simulink model "loadSimulator"  (R2025b)
settings: Solver=VariableStepAuto  StartTime=0.0  StopTime=50  RelTol=1e-3
values from neighbouring files (symbols this model uses):
  xL0 = [0.8;0.8;0.1]    [parametrosCarga4x.m]
settings Model: Creator=ateveraz  LastModifiedBy=ateveraz

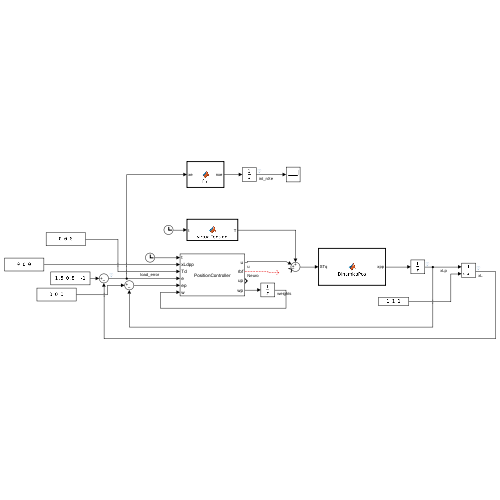
[thumbnail: Simulink's stored preview of the top-level diagram]
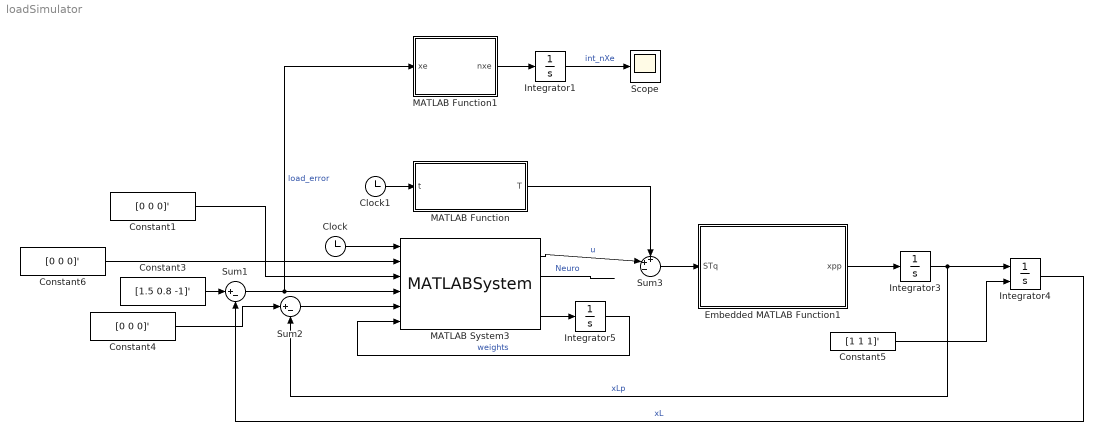
== system loadSimulator ==
  Clock : Clock
  Clock1 : Clock
  Constant1 : Constant  Value=[0 0 0]'
  Constant3 : Constant  Value=[1.5 0.8 -1]'
  Constant4 : Constant  Value=[0 0 0]'
  Constant5 : Constant  Value=[1 1 1]'
  Constant6 : Constant  Value=[0 0 0]'
  Embedded MATLAB Function1 : MATLAB Function  TreatAsAtomicUnit=on
  Integrator1 : Integrator
  Integrator3 : Integrator  InitFcn=parametrosCarga4x  InitialCondition=[0;0;0]
  Integrator4 : Integrator  InitFcn=parametrosCarga4x  InitialConditionSource=external  InitialCondition=xL0
  Integrator5 : Integrator  InitialCondition=zeros(3,15)
  MATLAB Function : MATLAB Function  TreatAsAtomicUnit=on
  MATLAB Function1 : MATLAB Function  TreatAsAtomicUnit=on
  MATLAB System3 : MATLABSystem  System=PositionController  Kd=2.0  alpha=1.0  mass=-0.225  Gamma=0.1  kappa=0.01  k=10  N_neurons=15  center_range=1.0  eta_width=1.5  SimulateUsing=Code generation
      mask Type: PositionController
  Scope : Scope
      settings: ActiveDisplayYMinimum=-1  ActiveDisplayYMaximum=1
  Sum1 : Sum  Inputs=|+-
  Sum2 : Sum  Inputs=|+-
  Sum3 : Sum  Inputs=++-|
  wires:
  Constant3/1 -> Sum1/1
  Sum1/1 -> MATLAB Function1/1(xe), MATLAB System3/4  "load_error"
  Sum2/1 -> MATLAB System3/5
  Constant4/1 -> Sum2/1
  Embedded MATLAB Function1/1(xpp) -> Integrator3/1
  Constant5/1 -> Integrator4/2
  Integrator3/1 -> Integrator4/1, Sum2/2  "xLp"
  Integrator4/1 -> Sum1/2  "xL"
  Sum3/1 -> Embedded MATLAB Function1/1(STq)
  MATLAB System3/2 -> ?  "Neuro"
  MATLAB System3/1 -> Sum3/2  "u"
  Constant6/1 -> MATLAB System3/2
  Clock/1 -> MATLAB System3/1
  MATLAB System3/4 -> Integrator5/1
  Integrator5/1 -> MATLAB System3/6  "weights"
  Constant1/1 -> MATLAB System3/3
  Clock1/1 -> MATLAB Function/1(t)
  MATLAB Function/1(T) -> Sum3/1
  MATLAB Function1/1(nxe) -> Integrator1/1
  Integrator1/1 -> Scope/1  "int_nXe"

== matlab function loadSimulator/Embedded MATLAB Function1 ==
  settings: updateMethod=CONTINUOUS  sampleTime=0.025
  data: STq input; xpp output
function xpp = DinamicaPos(STq)
%% Datos Dinámica
 mL = 0.225;
ez = [0;0;1];
g = 9.81*ez;

%% Dinámica
xpp = -STq/mL-g;

end

== matlab function loadSimulator/MATLAB Function ==
  data: t input; T output
function T = virtualTension(t)
    T = zeros(3,1);

    if (t > 20 && t < 30)
        a = 0.5;
        T(1) = a * cos(t-20);
        T(2) = -a * sin(t-20);
        T(3) = a * cos(2*t);
    end
end

== matlab function loadSimulator/MATLAB Function1 ==
  data: xe input; nxe output
function nxe  = fcn(xe)
    nxe = norm(xe);
end
